simulink model "MBD_Week2_Prob3"  (R2020a)
settings: Solver=VariableStepAuto  StartTime=0.0  StopTime=10.0  RelTol=1e-3
undefined symbols (not defined in the file or in its folder): b, m
settings Model: DataDictionary=DD_Cruise_Control.sldd  Creator=Noel Varghese  LastModifiedBy=Noel Varghese

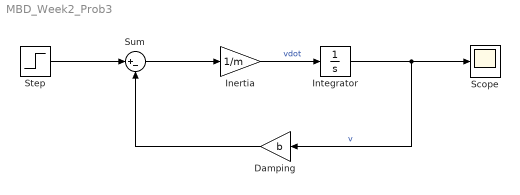
== system MBD_Week2_Prob3 ==
  Damping : Gain  Gain=b
  Inertia : Gain  Gain=1/m
  Integrator : Integrator
  Scope : Scope
  Step : Step  After=u  SampleTime=0
  Sum : Sum  Inputs=|+-
  wires:
  Inertia/1 -> Integrator/1  "vdot"
  Integrator/1 -> Scope/1, Damping/1  "v"
  Sum/1 -> Inertia/1
  Damping/1 -> Sum/2
  Step/1 -> Sum/1
